simulink model "gantrycrane_sim"  (Simulink 8.3)
settings: Solver=ode45  StartTime=0.0  StopTime=60  RelTol=1e-3
undefined symbols (not defined in the file or in its folder): crane_ctrlss, drawGantryCrane, P
libraries: simulink x1
settings Model: Creator=nedward  LastModifiedBy=jhl48
settings OptimizationCC: ExpressionDepthLimit=2147483647
settings DebuggingCC: FcnCallInpInsideContextMsg=UseLocalSettings

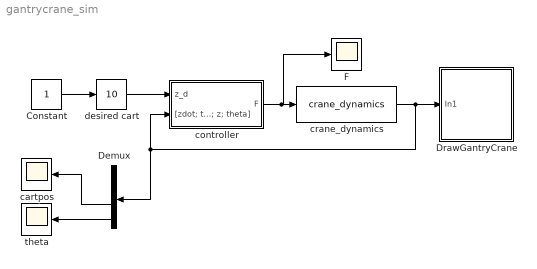
== system gantrycrane_sim ==
  Constant : Constant
  Demux : Demux
  DrawGantryCrane : Subsystem
      mask init:
      | bar = 20;
      | crane = [5 3];
      | L1 = 10;
      | R1 = 1;
      mask Display: image(imread('tv.jpg'))
  F : Scope
      settings: TimeRange=30  YMin=-20000  YMax=20000  SaveName=ScopeData3
  cartpos : Scope
      settings: TimeRange=30  YMin=-0.35  YMax=-0.18
  controller : Subsystem
  crane_dynamics : S-Function  FunctionName=crane_dynamics  Parameters=P  EnableBusSupport=off
  desired cart : simulink/Math Operations/Slider Gain  low=-10  gain=10  high=10
  theta : Scope
      settings: TimeRange=30  YMin=-3  YMax=3
  wires:
  crane_dynamics/1 -> controller/2("[zdot; thetadot; z; theta]"), Demux/1, DrawGantryCrane/1(In1)
  Constant/1 -> desired cart/1
  controller/1(F) -> F/1, crane_dynamics/1
  Demux/4 -> theta/1
  Demux/3 -> cartpos/1
  desired cart/1 -> controller/1(z_d)

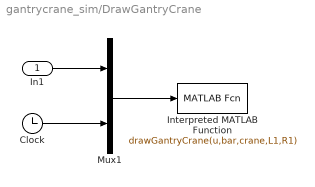
== system gantrycrane_sim/DrawGantryCrane ==
  In1 : Inport
  Clock : Clock
  Interpreted MATLAB Function : MATLABFcn  MATLABFcn=drawGantryCrane(u,bar,crane,L1,R1)  OutputDimensions=0  SampleTime=0.1
  Mux1 : Mux  Inputs=2
  wires:
  Clock/1 -> Mux1/2
  Mux1/1 -> Interpreted MATLAB Function/1
  In1/1 -> Mux1/1

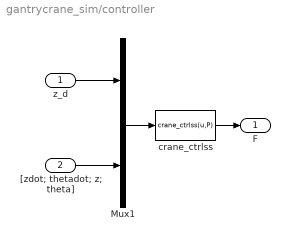
== system gantrycrane_sim/controller ==
  z_d : Inport
  "[zdot; thetadot; z; theta]" : Inport  Port=2
  Mux1 : Mux  Inputs=2
  crane_ctrlss : MATLABFcn  MATLABFcn=crane_ctrlss(u,P)  OutputDimensions=1  SampleTime=P.Ts
  F : Outport
  wires:
  crane_ctrlss/1 -> F/1
  "[zdot; thetadot; z; theta]"/1 -> Mux1/2
  z_d/1 -> Mux1/1
  Mux1/1 -> crane_ctrlss/1
